simulink subsystem "mechtoelecpower"  (R2022b)
settings: Solver=VariableStepAuto  StartTime=0.0  StopTime=10.0  RelTol=1e-3
settings Model: Creator=serga  LastModifiedBy=serga

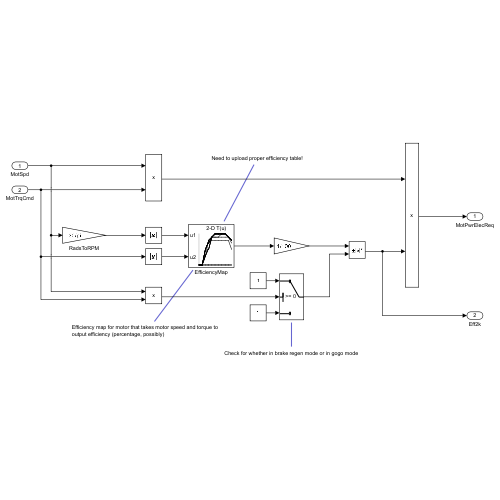
[thumbnail: Simulink's stored preview of the top-level diagram]
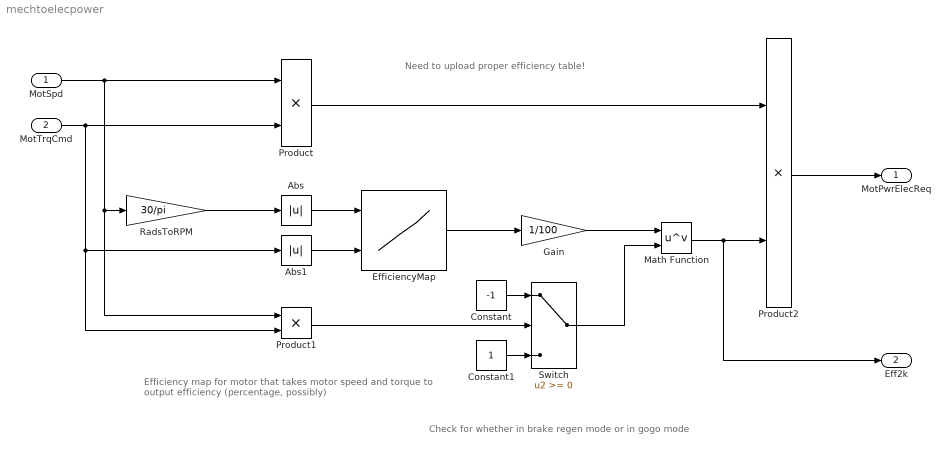
== system mechtoelecpower ==
  note: Need to upload proper efficiency table!
  note: Check for whether in brake regen mode or in gogo mode
  note: Efficiency map for motor that takes motor speed and torque to output efficiency (percentage, possibly)
  MotSpd : Inport
  MotTrqCmd : Inport  Port=2
  Abs : Abs  SaturateOnIntegerOverflow=off
  Abs1 : Abs  SaturateOnIntegerOverflow=off
  Constant : Constant  Value=-1
  Constant1 : Constant
  EfficiencyMap : Lookup_n-D  BreakpointsForDimension1=[0;1600;3200;4477.56;4800;6400;8000;9600;11200;12800;14400;16000]  BreakpointsForDimension2=[0 32.1428571428571 64.2857142857143 96.4285714285714 128.571428571429 160.714285714286 192.857142857143 225 257.142857142857 289.285714285714 321.428571428571 353.571428571429 385.714285714286 417.857142857143 450]  Table=[86.7 86.7 86.7 86.7 86.7 86.7 86.7 86.7 86.7 86.7 86.7 86.7 86.7 86.7 86.7;86.7 86.7 86.7 86.7 86.7 86.7 86.7 86.7 86.7 86.7 86.7 86.7 86.7 86.7 86.7;86.7 86.7 91.8 91.8 91.8 91.8 91.8 91.8 91.8 91.8 89.76 89.76 89.76 89.76 89.76;86.7 86.7 93.84 93.84 93.84 93.84 93.84 93.84 93.84 93.84 93.84 91.8 91.8 91.8 91.8;86.7 86.7 93.84 93.84 94.86 94.86 94.86 94.86 93.84 93.84 93.84 91.8 91.8 91.8 91.8;86.7 86.7 94.86 95.88 95.88 95.88 95.88 95.88 95.88 95.88 95.88 95.88 95.88 95.88 95.88;86.7 86.7 94.86 95.88 95.88 96.9 96.9 96.9 96.9 96.9 96.9 96.9 96.9 96.9 96.9;86.7 86.7 94.86 95.88 95.88 96.9 96.9 96.9 96.9 96.9 96.9 96.9 96.9 96.9 96.9;86.7 86.7 94.86 95.88 96.9 96.9 96.9 96.9 96.9 96.9 96.9 96.9 96.9 96.9 96.9;86.7 86.7 94.86 95.88 96.9 96.9 96.9 96.9 96.9 96.9 96.9 96.9 96.9 96.9 96.9;86.7 86.7 94.86 95.88 95.88 95.88 95.88 95.88 95.88 95.88 95.88 95.88 95.88 95.88 95.88;86.7 86.7 91.8 93.84 94.86 94.86 94.86 94.86 94.86 94.86 94.86 94.86 94.86 94.86 94.86]  ExtrapMethod=Clip  UseLastTableValue=on  InternalRulePriority=Speed  OutDataTypeStr=Inherit: Inherit from 'Table data'  RndMeth=Simplest
      settings: InputPortMap=u0,u1
  Gain : Gain  Gain=1/100
  Math Function : Math  Operator=pow  SignedPower=on  OutputSignalType=real
  Product : Product
  Product1 : Product
  Product2 : Product
  RadsToRPM : Gain  Gain=30/pi
  Switch : Switch  SaturateOnIntegerOverflow=off  InputSameDT=off
  MotPwrElecReq : Outport
  Eff2k : Outport  Port=2
  wires:
  MotSpd/1 -> RadsToRPM/1, Product1/1, Product/1
  MotTrqCmd/1 -> Product1/2, Abs1/1, Product/2
  RadsToRPM/1 -> Abs/1
  Abs/1 -> EfficiencyMap/1
  Abs1/1 -> EfficiencyMap/2
  Product1/1 -> Switch/2
  Constant1/1 -> Switch/3
  Constant/1 -> Switch/1
  EfficiencyMap/1 -> Gain/1
  Switch/1 -> Math Function/2
  Gain/1 -> Math Function/1
  Math Function/1 -> Eff2k/1, Product2/2
  Product/1 -> Product2/1
  Product2/1 -> MotPwrElecReq/1
